simulink model "TDPBehaviourSim"  (R2020b)
settings: Solver=VariableStepAuto  StartTime=0.0  StopTime=200  FixedStep=sampleTime  RelTol=1e-3  EnableMultiTasking=on
values from neighbouring files (symbols this model uses):
  angThresh = pi/16    (= 0.196349540849)    [GameParameters.m]
  attackerKickSpeed = 0.3    [GameParameters.m]
  AwayFormation1 = [9.5 4 pi ... (first row only)    [FormationPoses.m]    (also in GameParameters.m)
  ballAngleNoise = pi/24    (= 0.1308996939)    [GameParameters.m]
  ballThresh = playerRadius + 0.03    (= 0.11)    [GameParameters.m]
  ballVelNoise = 0.05    [GameParameters.m]
  distThresh = 0.1    [GameParameters.m]
  fieldCenter = [mean(fieldLimitsX) mean(fieldLimitsY)]    [GameParameters.m]
  fieldLimitsX = [1 10]    [GameParameters.m]
  fieldLimitsY = [1 7]    [GameParameters.m]
  goalPosts = [1  2.7 2 ... (first row only)    [GameParameters.m]
  HomeFormation1 = [1.5 4 0 ... (first row only)    [FormationPoses.m]    (also in GameParameters.m)
  maxSpeed = 0.1    [GameParameters.m]
  maxTurnSpeed = 0.05    [GameParameters.m]
  playerRadius = 0.08    [GameParameters.m]
  sampleTime = 0.5    [GameParameters.m]
undefined symbols (not defined in the file or in its folder): DiscIntNeverNeededParam
libraries: mobileRoboticsLib x33, soccerRobotLib x16
(part 1 of 2)
settings Model: SimulationMode=accelerator  SnapshotBufferSize=20  Creator=2683935i  LastModifiedBy=2683935i
settings SolverCC: AutoInsertRateTranBlk=on
settings DataIOCC: SaveOutput=off  SaveTime=off
settings OptimizationCC: DefaultParameterBehavior=Inlined  InlineInvariantSignals=on  EnhancedBackFolding=on  PassReuseOutputArgsAs=Individual arguments  StateBitsets=on  DataBitsets=on  ZeroExternalMemoryAtStartup=off  ZeroInternalMemoryAtStartup=off  NoFixptDivByZeroProtection=on  LifeSpan=1  OptimizeBlockOrder=speed  DifferentSizesBufferReuse=on  EfficientTunableParamExpr=on
settings DebuggingCC: ParameterTunabilityLossMsg=error  UnderSpecifiedDimensionMsg=warning
settings HardwareCC: ProdBitPerPointer=32  ProdBitPerSizeT=32  ProdBitPerPtrDiffT=32  ProdLargestAtomicFloat=None  ProdIntDivRoundTo=Floor  ProdWordSize=32  ProdHWDeviceType=Generic->Custom
settings SFSimCC: MATLABDynamicMemAlloc=off
settings RTWCC: Description=Embedded Coder  SystemTargetFile=ert.tlc  TLCOptions=-p0  GenCodeOnly=on  TemplateMakefile=ert_default_tmf  GenerateReport=on  RTWVerbose=off  IncludeHyperlinkInReport=on  LaunchReport=on
settings CodeAppCC: ForceParamTrailComments=on  IgnoreCustomStorageClasses=off  OperatorAnnotations=on  SimulinkDataObjDesc=on  SFDataObjDesc=on  CustomSymbolStrGlobalVar=rt$N$M  CustomSymbolStrType=$N$M  CustomSymbolStrFcn=$N$M$F  CustomSymbolStrMacro=$N$M  InsertBlockDesc=on
settings ERTTargetCC: TargetLangStandard=C99 (ISO)  GenerateSampleERTMain=on  IncludeMdlTerminateFcn=off  SuppressErrorStatus=on  SupportAbsoluteTime=off  PurelyIntegerCode=on  SupportNonFinite=off  SupportComplex=off  InlinedParameterPlacement=NonHierarchical  RootIOFormat=Structure reference  ERTCustomFileTemplate=example_file_process.tlc

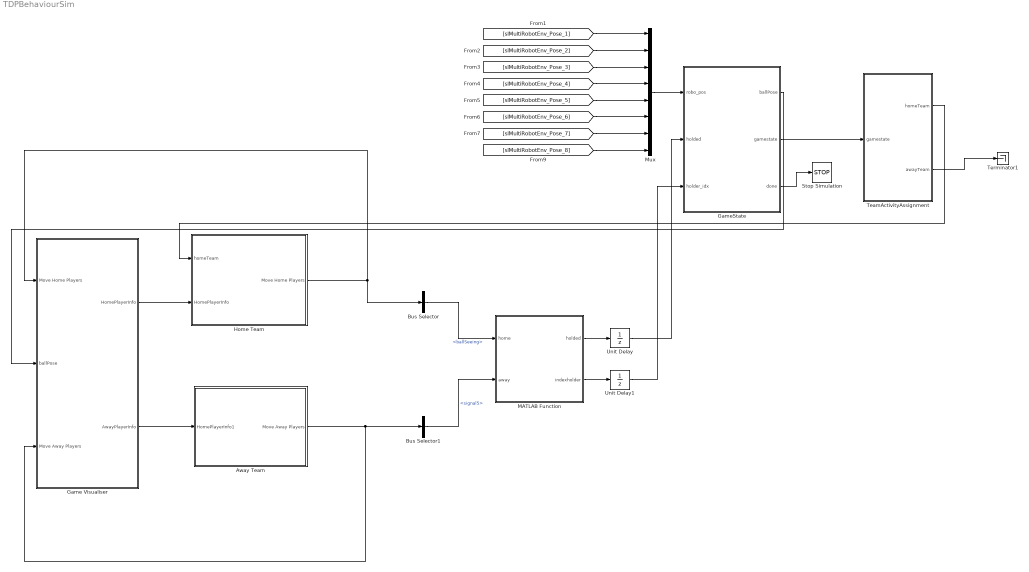
== system TDPBehaviourSim ==
  Away Team : Subsystem
  Bus Selector : BusSelector  OutputSignals=ballSeeing
  Bus Selector1 : BusSelector  OutputSignals=signal5
  Game Visualiser : Subsystem
  GameState : Stateflow chart  TreatAsAtomicUnit=on
  Home Team : Subsystem
  MATLAB Function : MATLAB Function  TreatAsAtomicUnit=on
  Mux : Mux  Inputs=8
  Stop Simulation : Stop
  TeamActivityAssignment : Stateflow chart  TreatAsAtomicUnit=on
  Terminator1 : Terminator
  Unit Delay : UnitDelay  SampleTime=-1  HasFrameUpgradeWarning=on
  Unit Delay1 : UnitDelay  SampleTime=-1  HasFrameUpgradeWarning=on
  wires:
  Home Team/1(Move Home Players) -> Bus Selector/1, Game Visualiser/1(Move Home Players)
  Away Team/1(Move Away Players) -> Game Visualiser/3(Move Away Players), Bus Selector1/1
  Game Visualiser/1(HomePlayerInfo) -> Home Team/2(HomePlayerInfo)
  Game Visualiser/2(AwayPlayerInfo) -> Away Team/1(HomePlayerInfo1)
  [slMultiRobotEnv_Pose_4] -> Mux/4
  [slMultiRobotEnv_Pose_8] -> Mux/8
  [slMultiRobotEnv_Pose_1] -> Mux/1
  Mux/1 -> GameState/1(robo_pos)
  [slMultiRobotEnv_Pose_2] -> Mux/2
  [slMultiRobotEnv_Pose_3] -> Mux/3
  GameState/1(ballPose) -> Game Visualiser/2(ballPose)
  TeamActivityAssignment/2(awayTeam) -> Terminator1/1
  TeamActivityAssignment/1(homeTeam) -> Home Team/1(homeTeam)
  Bus Selector/1 -> MATLAB Function/1(home)  "<ballSeeing>"
  Bus Selector1/1 -> MATLAB Function/2(away)  "<signal5>"
  GameState/3(done) -> Stop Simulation/1
  [slMultiRobotEnv_Pose_5] -> Mux/5
  [slMultiRobotEnv_Pose_6] -> Mux/6
  [slMultiRobotEnv_Pose_7] -> Mux/7
  GameState/2(gamestate) -> TeamActivityAssignment/1(gamestate)
  MATLAB Function/2(indexholder) -> Unit Delay1/1
  Unit Delay1/1 -> GameState/3(holder_idx)
  MATLAB Function/1(holded) -> Unit Delay/1
  Unit Delay/1 -> GameState/2(holded)

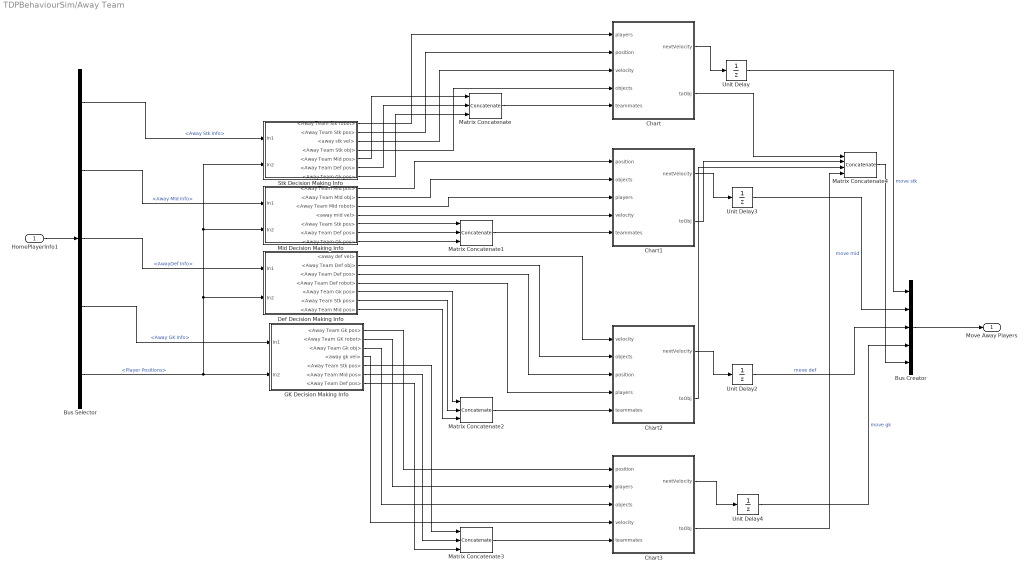
== system TDPBehaviourSim/Away Team ==
  HomePlayerInfo1 : Inport
  Bus Creator : BusCreator  Inputs=5
  Bus Selector : BusSelector  OutputSignals=Away Stk Info,Away MId Info,AwayDef Info,Away GK Info,Player Positions
  Chart : Stateflow chart  TreatAsAtomicUnit=on
      settings: PortSchema="{\"entries\":[{\"content\":{\"sides\":[{\"content\":{\"connectorIds\":[\"In3\",\"In1\",\"In2\",\"In5\",\"In4\"]},\"type\":\"ConnectorPlacement.EquallySpacedRectSide\",\"uuid\":\"cf890ef0-0ec1-422c-ab9c-1628c873ebf0\"},{\"content\":{\"connectorIds\":[\"Out1\",\"Out2\"],\"side\":\"RIGHT\"},\"type\":\"ConnectorPlacement.EquallySpacedRectSide\",\"uuid\":\"0000e457-9393-40de-9950-8ff794b83dda\"},{\"content\":{\"connectorIds\":[],\"side\":\"TOP\"},\"type\":\"ConnectorPlacement.EquallySpacedRectSide\",\"uuid\":\"7dd8e30a-3952-4d7c-b255-0e0c48dee19a\"}]},\"type\":\"ConnectorPlacement.EquallySpacedConnector\",\"uuid\":\"e8168788-1535-41f0-a84f-110f92e839bd\"}],\"packageUris\":[\"http://schema.mathworks.com/mf0/Connector/R2020b\"],\"version\":\"1.0\"}"
  Chart1 : Stateflow chart  TreatAsAtomicUnit=on
      settings: PortSchema="{\"entries\":[{\"content\":{\"sides\":[{\"content\":{\"connectorIds\":[\"In1\",\"In5\",\"In3\",\"In2\",\"In4\"]},\"type\":\"ConnectorPlacement.EquallySpacedRectSide\",\"uuid\":\"cf890ef0-0ec1-422c-ab9c-1628c873ebf0\"},{\"content\":{\"connectorIds\":[\"Out1\",\"Out2\"],\"side\":\"RIGHT\"},\"type\":\"ConnectorPlacement.EquallySpacedRectSide\",\"uuid\":\"0000e457-9393-40de-9950-8ff794b83dda\"},{\"content\":{\"connectorIds\":[],\"side\":\"TOP\"},\"type\":\"ConnectorPlacement.EquallySpacedRectSide\",\"uuid\":\"7dd8e30a-3952-4d7c-b255-0e0c48dee19a\"}]},\"type\":\"ConnectorPlacement.EquallySpacedConnector\",\"uuid\":\"e8168788-1535-41f0-a84f-110f92e839bd\"}],\"packageUris\":[\"http://schema.mathworks.com/mf0/Connector/R2020b\"],\"version\":\"1.0\"}"
  Chart2 : Stateflow chart  TreatAsAtomicUnit=on
      settings: PortSchema="{\"entries\":[{\"content\":{\"sides\":[{\"content\":{\"connectorIds\":[\"In2\",\"In5\",\"In1\",\"In3\",\"In4\"]},\"type\":\"ConnectorPlacement.EquallySpacedRectSide\",\"uuid\":\"cf890ef0-0ec1-422c-ab9c-1628c873ebf0\"},{\"content\":{\"connectorIds\":[\"Out1\",\"Out2\"],\"side\":\"RIGHT\"},\"type\":\"ConnectorPlacement.EquallySpacedRectSide\",\"uuid\":\"0000e457-9393-40de-9950-8ff794b83dda\"},{\"content\":{\"connectorIds\":[],\"side\":\"TOP\"},\"type\":\"ConnectorPlacement.EquallySpacedRectSide\",\"uuid\":\"7dd8e30a-3952-4d7c-b255-0e0c48dee19a\"}]},\"type\":\"ConnectorPlacement.EquallySpacedConnector\",\"uuid\":\"e8168788-1535-41f0-a84f-110f92e839bd\"}],\"packageUris\":[\"http://schema.mathworks.com/mf0/Connector/R2020b\"],\"version\":\"1.0\"}"
  Chart3 : Stateflow chart  TreatAsAtomicUnit=on
      settings: PortSchema="{\"entries\":[{\"content\":{\"sides\":[{\"content\":{\"connectorIds\":[\"In1\",\"In3\",\"In5\",\"In2\",\"In4\"]},\"type\":\"ConnectorPlacement.EquallySpacedRectSide\",\"uuid\":\"cf890ef0-0ec1-422c-ab9c-1628c873ebf0\"},{\"content\":{\"connectorIds\":[\"Out1\",\"Out2\"],\"side\":\"RIGHT\"},\"type\":\"ConnectorPlacement.EquallySpacedRectSide\",\"uuid\":\"0000e457-9393-40de-9950-8ff794b83dda\"},{\"content\":{\"connectorIds\":[],\"side\":\"TOP\"},\"type\":\"ConnectorPlacement.EquallySpacedRectSide\",\"uuid\":\"7dd8e30a-3952-4d7c-b255-0e0c48dee19a\"}]},\"type\":\"ConnectorPlacement.EquallySpacedConnector\",\"uuid\":\"e8168788-1535-41f0-a84f-110f92e839bd\"}],\"packageUris\":[\"http://schema.mathworks.com/mf0/Connector/R2020b\"],\"version\":\"1.0\"}"
  Def Decision Making Info : Subsystem
  GK Decision Making Info : Subsystem
  Matrix Concatenate{,1..3} (4 alike) : Concatenate  NumInputs=3  Mode=Multidimensional array  ConcatenateDimension=2
  Matrix Concatenate4 : Concatenate  NumInputs=4  Mode=Multidimensional array
  Mid Decision Making Info : Subsystem
  Stk Decision Making Info : Subsystem
  Unit Delay{,2..4} (4 alike) : UnitDelay  SampleTime=-1  HasFrameUpgradeWarning=on
  Move Away Players : Outport
  wires:
  Def Decision Making Info/7(<Away Team Mid pos>) -> Matrix Concatenate2/3
  Def Decision Making Info/6(<Away Team Stk pos>) -> Matrix Concatenate2/2
  Def Decision Making Info/3(<Away Team Def pos>) -> Chart2/1(position)
  Matrix Concatenate3/1 -> Chart3/4(teammates)
  Unit Delay/1 -> Bus Creator/1  "move stk"
  Stk Decision Making Info/6(<Away Team Def pos>) -> Matrix Concatenate/2
  Stk Decision Making Info/5(<Away Team Mid pos>) -> Matrix Concatenate/1
  Mid Decision Making Info/6(<Away Team Def pos>) -> Matrix Concatenate1/2
  Def Decision Making Info/1(<away def vel>) -> Chart2/2(velocity)
  Mid Decision Making Info/1(<Away Team Mid pos>) -> Chart1/1(position)
  Mid Decision Making Info/7(<Away Team Gk pos>) -> Matrix Concatenate1/3
  Mid Decision Making Info/4(<away mid vel>) -> Chart1/2(velocity)
  GK Decision Making Info/7(<Away Team Def pos>) -> Matrix Concatenate3/3
  GK Decision Making Info/2(<Away Team GK robot>) -> Chart3/3(players)
  GK Decision Making Info/1(<Away Team Gk pos>) -> Chart3/1(position)
  Matrix Concatenate/1 -> Chart/4(teammates)
  Stk Decision Making Info/4(<Away Team Stk obj>) -> Chart/5(objects)
  Chart1/1(nextVelocity) -> Unit Delay3/1
  Mid Decision Making Info/2(<Away Team MId obj>) -> Chart1/5(objects)
  Chart2/1(nextVelocity) -> Unit Delay2/1
  Mid Decision Making Info/3(<Away Team MId robot>) -> Chart1/3(players)
  GK Decision Making Info/6(<Away Team Mid pos>) -> Matrix Concatenate3/2
  Chart/1(nextVelocity) -> Unit Delay/1
  Unit Delay4/1 -> Bus Creator/4  "move gk"
  Mid Decision Making Info/5(<Away Team Stk pos>) -> Matrix Concatenate1/1
  Def Decision Making Info/2(<Away Team Def obj>) -> Chart2/5(objects)
  Stk Decision Making Info/1(<Away Team Stk robot>) -> Chart/3(players)
  Def Decision Making Info/4(<Away Team Def robot>) -> Chart2/3(players)
  Chart3/1(nextVelocity) -> Unit Delay4/1
  Matrix Concatenate1/1 -> Chart1/4(teammates)
  GK Decision Making Info/3(<Away Team Gk obj>) -> Chart3/5(objects)
  Stk Decision Making Info/3(<away stk vel>) -> Chart/2(velocity)
  GK Decision Making Info/4(<away gk vel>) -> Chart3/2(velocity)
  Stk Decision Making Info/2(<Away Team Stk pos>) -> Chart/1(position)
  Matrix Concatenate2/1 -> Chart2/4(teammates)
  Stk Decision Making Info/7(<Away Team Gk pos>) -> Matrix Concatenate/3
  Def Decision Making Info/5(<Away Team Gk pos>) -> Matrix Concatenate2/1
  Unit Delay2/1 -> Bus Creator/3  "move def"
  GK Decision Making Info/5(<Away Team Stk pos>) -> Matrix Concatenate3/1
  Unit Delay3/1 -> Bus Creator/2  "move mid"
  Bus Creator/1 -> Move Away Players/1
  HomePlayerInfo1/1 -> Bus Selector/1
  Bus Selector/5 -> Stk Decision Making Info/2(In2), Mid Decision Making Info/2(In2), Def Decision Making Info/2(In2), GK Decision Making Info/2(In2)  "<Player Positions>"
  Bus Selector/1 -> Stk Decision Making Info/1(In1)  "<Away Stk Info>"
  Bus Selector/2 -> Mid Decision Making Info/1(In1)  "<Away MId Info>"
  Bus Selector/3 -> Def Decision Making Info/1(In1)  "<AwayDef Info>"
  Bus Selector/4 -> GK Decision Making Info/1(In1)  "<Away GK Info>"
  Chart/2(toObj) -> Matrix Concatenate4/1
  Chart1/2(toObj) -> Matrix Concatenate4/2
  Chart2/2(toObj) -> Matrix Concatenate4/3
  Chart3/2(toObj) -> Matrix Concatenate4/4
  Matrix Concatenate4/1 -> Bus Creator/5

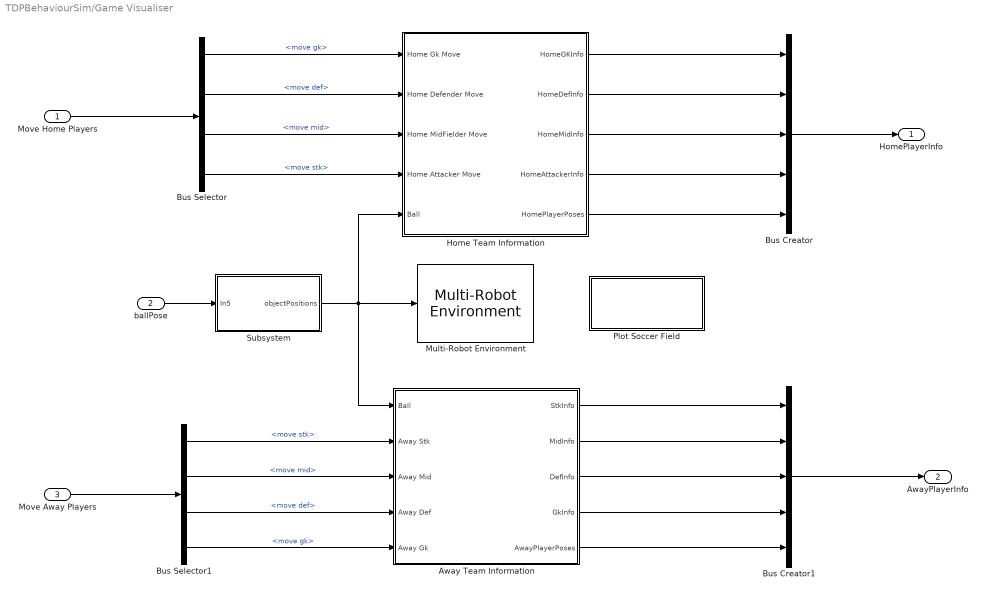
== system TDPBehaviourSim/Game Visualiser ==
  Move Home Players : Inport
  ballPose : Inport  Port=2
  Move Away Players : Inport  Port=3
  Away Team Information : Subsystem
  Bus Creator : BusCreator  Inputs=5
  Bus Creator1 : BusCreator  Inputs=5
  Bus Selector : BusSelector  OutputSignals=move gk,move def,move mid,move stk
  Bus Selector1 : BusSelector  OutputSignals=move stk,move mid,move def,move gk
  Home Team Information : Subsystem
  Multi-Robot Environment : mobileRoboticsLib/Environments/Multi-Robot Environment  numRobots=numPlayers  mapName=map  showWaypoints=off  showObjects=on  objectColors=objColors  objectMarkers='o^^^^'  showRobotIds=on  plotSensorLines=off
      settings: SourceProductName=Mobile Robotics Simulation Toolbox
  Plot Soccer Field : MATLAB Function  TreatAsAtomicUnit=on
  Subsystem : Subsystem
  HomePlayerInfo : Outport
  AwayPlayerInfo : Outport  Port=2
  wires:
  Home Team Information/1(HomeGKInfo) -> Bus Creator/1
  Home Team Information/2(HomeDefInfo) -> Bus Creator/2
  Home Team Information/3(HomeMidInfo) -> Bus Creator/3
  Home Team Information/4(HomeAttackerInfo) -> Bus Creator/4
  Home Team Information/5(HomePlayerPoses) -> Bus Creator/5
  Away Team Information/1(StkInfo) -> Bus Creator1/1
  Away Team Information/2(MidInfo) -> Bus Creator1/2
  Away Team Information/3(DefInfo) -> Bus Creator1/3
  Away Team Information/4(GkInfo) -> Bus Creator1/4
  Away Team Information/5(AwayPlayerPoses) -> Bus Creator1/5
  Subsystem/1(objectPositions) -> Multi-Robot Environment/1, Away Team Information/1(Ball), Home Team Information/5(Ball)
  ballPose/1 -> Subsystem/1(In5)
  Move Home Players/1 -> Bus Selector/1
  Bus Selector/1 -> Home Team Information/1(Home Gk Move)  "<move gk>"
  Bus Selector/2 -> Home Team Information/2(Home Defender Move)  "<move def>"
  Bus Selector/3 -> Home Team Information/3(Home MidFielder Move)  "<move mid>"
  Bus Selector/4 -> Home Team Information/4(Home Attacker Move)  "<move stk>"
  Move Away Players/1 -> Bus Selector1/1
  Bus Selector1/4 -> Away Team Information/5("Away Gk ")  "<move gk>"
  Bus Selector1/3 -> Away Team Information/4(Away Def)  "<move def>"
  Bus Selector1/2 -> Away Team Information/3(Away Mid)  "<move mid>"
  Bus Selector1/1 -> Away Team Information/2(Away Stk)  "<move stk>"
  Bus Creator/1 -> HomePlayerInfo/1
  Bus Creator1/1 -> AwayPlayerInfo/1

== system TDPBehaviourSim/GameState/BallDynamics.InBounds.BallFree ==
  Action Port : ActionPort
      settings: CopyFcn=Stateflow.SLINSF.SimulinkMan.removeBlockPreDeleteFcn  PreDeleteFcn=Stateflow.SLINSF.SimulinkMan.unsafePredeleteFcn
  Gain : Gain  Gain=-0.25
  Position Integrator : DiscreteIntegrator  InitialCondition=fieldCenter  SampleTime=-1  StateName=ballPos  ICPrevOutput=DiscIntNeverNeededParam  ICPrevScaledInput=DiscIntNeverNeededParam
  Signal Specification : SignalSpecification  Dimensions=[1 2]
  Velocity Integrator : DiscreteIntegrator  InitialCondition=[0 0]  SampleTime=-1  StateName=ballVel  ICPrevOutput=DiscIntNeverNeededParam  ICPrevScaledInput=DiscIntNeverNeededParam
  ballPose : Outport  VectorParamsAs1DForOutWhenUnconnected=off
  wires:
  Gain/1 -> Velocity Integrator/1
  Velocity Integrator/1 -> Signal Specification/1
  Position Integrator/1 -> ballPose/1
  Signal Specification/1 -> Position Integrator/1, Gain/1

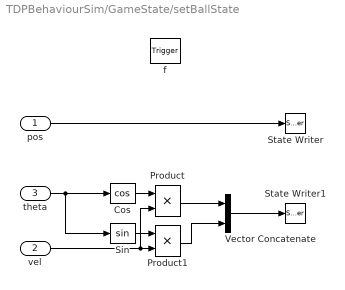
== system TDPBehaviourSim/GameState/setBallState ==
  pos : Inport  OutDataTypeStr=double  PortDimensions=[1 2]
  vel : Inport  Port=2  OutDataTypeStr=double  PortDimensions=1
  theta : Inport  Port=3  OutDataTypeStr=double  PortDimensions=1
  f : TriggerPort  TriggerType=function-call  VariantControl=(inherit)
      settings: CopyFcn=Stateflow.SLINSF.SimulinkMan.removeBlockPreDeleteFcn  PreDeleteFcn=Stateflow.SLINSF.SimulinkMan.unsafePredeleteFcn
  Cos : Trigonometry  Operator=cos
  Product : Product
  Product1 : Product
  Sin : Trigonometry
  State Writer : StateWriter  StateOwnerBlock=../../BallDynamics.InBounds.BallFree/Position Integrator  StateName=ballPos
  State Writer1 : StateWriter  StateOwnerBlock=../../BallDynamics.InBounds.BallFree/Velocity Integrator  StateName=ballVel
  Vector Concatenate : Concatenate  Mode=Multidimensional array  ConcatenateDimension=2
  wires:
  Vector Concatenate/1 -> State Writer1/1
  Product1/1 -> Vector Concatenate/2
  Product/1 -> Vector Concatenate/1
  theta/1 -> Cos/1, Sin/1
  Sin/1 -> Product1/1
  vel/1 -> Product1/2, Product/2
  Cos/1 -> Product/1
  pos/1 -> State Writer/1

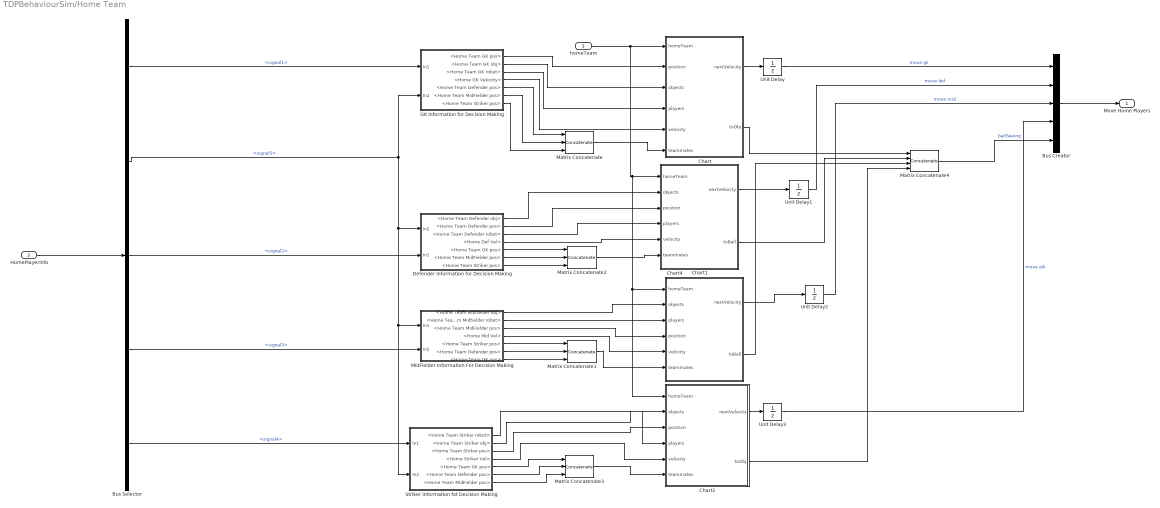
== system TDPBehaviourSim/Home Team ==
  homeTeam : Inport
  HomePlayerInfo : Inport  Port=2
  Bus Creator : BusCreator  Inputs=5
  Bus Selector : BusSelector  OutputSignals=signal1,signal5,signal2,signal3,signal4
  Chart : Stateflow chart  TreatAsAtomicUnit=on
      settings: PortSchema="{\"entries\":[{\"content\":{\"sides\":[{\"content\":{\"connectorIds\":[\"In1\",\"In2\",\"In6\",\"In4\",\"In3\",\"In5\"]},\"type\":\"ConnectorPlacement.EquallySpacedRectSide\",\"uuid\":\"cf890ef0-0ec1-422c-ab9c-1628c873ebf0\"},{\"content\":{\"connectorIds\":[\"Out1\",\"Out2\"],\"side\":\"RIGHT\"},\"type\":\"ConnectorPlacement.EquallySpacedRectSide\",\"uuid\":\"0000e457-9393-40de-9950-8ff794b83dda\"},{\"content\":{\"connectorIds\":[],\"side\":\"TOP\"},\"type\":\"ConnectorPlacement.EquallySpacedRectSide\",\"uuid\":\"7dd8e30a-3952-4d7c-b255-0e0c48dee19a\"}]},\"type\":\"ConnectorPlacement.EquallySpacedConnector\",\"uuid\":\"e8168788-1535-41f0-a84f-110f92e839bd\"}],\"packageUris\":[\"http://schema.mathworks.com/mf0/Connector/R2020b\"],\"version\":\"1.0\"}"
  Chart1 : Stateflow chart  TreatAsAtomicUnit=on
      settings: PortSchema="{\"entries\":[{\"content\":{\"sides\":[{\"content\":{\"connectorIds\":[\"In1\",\"In6\",\"In2\",\"In4\",\"In3\",\"In5\"]},\"type\":\"ConnectorPlacement.EquallySpacedRectSide\",\"uuid\":\"cf890ef0-0ec1-422c-ab9c-1628c873ebf0\"},{\"content\":{\"connectorIds\":[\"Out1\",\"Out2\"],\"side\":\"RIGHT\"},\"type\":\"ConnectorPlacement.EquallySpacedRectSide\",\"uuid\":\"0000e457-9393-40de-9950-8ff794b83dda\"},{\"content\":{\"connectorIds\":[],\"side\":\"TOP\"},\"type\":\"ConnectorPlacement.EquallySpacedRectSide\",\"uuid\":\"7dd8e30a-3952-4d7c-b255-0e0c48dee19a\"}]},\"type\":\"ConnectorPlacement.EquallySpacedConnector\",\"uuid\":\"e8168788-1535-41f0-a84f-110f92e839bd\"}],\"packageUris\":[\"http://schema.mathworks.com/mf0/Connector/R2020b\"],\"version\":\"1.0\"}"
  Chart2 : Stateflow chart  TreatAsAtomicUnit=on
      settings: PortSchema="{\"entries\":[{\"content\":{\"sides\":[{\"content\":{\"connectorIds\":[\"In1\",\"In6\",\"In2\",\"In4\",\"In3\",\"In5\"]},\"type\":\"ConnectorPlacement.EquallySpacedRectSide\",\"uuid\":\"cf890ef0-0ec1-422c-ab9c-1628c873ebf0\"},{\"content\":{\"connectorIds\":[\"Out1\",\"Out2\"],\"side\":\"RIGHT\"},\"type\":\"ConnectorPlacement.EquallySpacedRectSide\",\"uuid\":\"0000e457-9393-40de-9950-8ff794b83dda\"},{\"content\":{\"connectorIds\":[],\"side\":\"TOP\"},\"type\":\"ConnectorPlacement.EquallySpacedRectSide\",\"uuid\":\"7dd8e30a-3952-4d7c-b255-0e0c48dee19a\"}]},\"type\":\"ConnectorPlacement.EquallySpacedConnector\",\"uuid\":\"e8168788-1535-41f0-a84f-110f92e839bd\"}],\"packageUris\":[\"http://schema.mathworks.com/mf0/Connector/R2020b\"],\"version\":\"1.0\"}"
  Chart4 : Stateflow chart  TreatAsAtomicUnit=on
      settings: PortSchema="{\"entries\":[{\"content\":{\"sides\":[{\"content\":{\"connectorIds\":[\"In1\",\"In6\",\"In4\",\"In2\",\"In3\",\"In5\"]},\"type\":\"ConnectorPlacement.EquallySpacedRectSide\",\"uuid\":\"cf890ef0-0ec1-422c-ab9c-1628c873ebf0\"},{\"content\":{\"connectorIds\":[\"Out1\",\"Out2\"],\"side\":\"RIGHT\"},\"type\":\"ConnectorPlacement.EquallySpacedRectSide\",\"uuid\":\"0000e457-9393-40de-9950-8ff794b83dda\"},{\"content\":{\"connectorIds\":[],\"side\":\"TOP\"},\"type\":\"ConnectorPlacement.EquallySpacedRectSide\",\"uuid\":\"7dd8e30a-3952-4d7c-b255-0e0c48dee19a\"}]},\"type\":\"ConnectorPlacement.EquallySpacedConnector\",\"uuid\":\"e8168788-1535-41f0-a84f-110f92e839bd\"}],\"packageUris\":[\"http://schema.mathworks.com/mf0/Connector/R2020b\"],\"version\":\"1.0\"}"
  "Defender Information for Decision Making " : Subsystem
  GK Information for Decision Making : Subsystem
  Matrix Concatenate{,1..3} (4 alike) : Concatenate  NumInputs=3  Mode=Multidimensional array  ConcatenateDimension=2
  Matrix Concatenate4 : Concatenate  NumInputs=4  Mode=Multidimensional array
  MidFielder Information For Decision Making : Subsystem
  Striker Information fot Decision Making : Subsystem
  Unit Delay{,1..3} (4 alike) : UnitDelay  SampleTime=-1  HasFrameUpgradeWarning=on
  Move Home Players : Outport
  wires:
  "Defender Information for Decision Making "/7(<Home Team Striker pos>) -> Matrix Concatenate2/3
  Matrix Concatenate1/1 -> Chart4/5(teammates)
  Striker Information fot Decision Making/7(<Home Team MidFielder pos>) -> Matrix Concatenate3/3
  "Defender Information for Decision Making "/3(<Home Team Defender robot>) -> Chart1/4(players)
  GK Information for Decision Making/1(<Home Team GK pos>) -> Chart/2(position)
  GK Information for Decision Making/4(<Home GK Velocity>) -> Chart/3(velocity)
  Chart/1(nextVelocity) -> Unit Delay/1
  "Defender Information for Decision Making "/6(<Home Team MidFielder pos>) -> Matrix Concatenate2/2
  GK Information for Decision Making/7(<Home Team Striker pos>) -> Matrix Concatenate/3
  MidFielder Information For Decision Making/3(<Home Team MidFielder pos>) -> Chart4/2(position)
  GK Information for Decision Making/3(<Home Team GK robot>) -> Chart/4(players)
  "Defender Information for Decision Making "/1(<Home Team Defender obj>) -> Chart1/6(objects)
  "Defender Information for Decision Making "/4(<Home Def Vel>) -> Chart1/3(velocity)
  GK Information for Decision Making/5(<Home Team Defender pos>) -> Matrix Concatenate/1
  MidFielder Information For Decision Making/2(<Home Team Midfielder robot>) -> Chart4/4(players)
  GK Information for Decision Making/6(<Home Team MidFielder pos>) -> Matrix Concatenate/2
  Matrix Concatenate2/1 -> Chart1/5(teammates)
  Striker Information fot Decision Making/6(<Home Team Defender pos>) -> Matrix Concatenate3/2
  MidFielder Information For Decision Making/5(<Home Team Striker pos>) -> Matrix Concatenate1/1
  MidFielder Information For Decision Making/7(<Home Team GK pos>) -> Matrix Concatenate1/3
  GK Information for Decision Making/2(<Home Team GK obj>) -> Chart/6(objects)
  MidFielder Information For Decision Making/4(<Home Mid Vel>) -> Chart4/3(velocity)
  MidFielder Information For Decision Making/1(<Home Team Midfielder obj>) -> Chart4/6(objects)
  Striker Information fot Decision Making/5(<Home Team GK pos>) -> Matrix Concatenate3/1
  Unit Delay/1 -> Bus Creator/1  "move gk"
  MidFielder Information For Decision Making/6(<Home Team Defender pos>) -> Matrix Concatenate1/2
  "Defender Information for Decision Making "/2(<Home Team Defender pos>) -> Chart1/2(position)
  "Defender Information for Decision Making "/5(<Home Team GK pos>) -> Matrix Concatenate2/1
  Chart2/1(nextVelocity) -> Unit Delay3/1
  Unit Delay2/1 -> Bus Creator/3  "move mid"
  Unit Delay1/1 -> Bus Creator/2  "move def"
  Matrix Concatenate/1 -> Chart/5(teammates)
  Bus Creator/1 -> Move Home Players/1
  HomePlayerInfo/1 -> Bus Selector/1
  Bus Selector/1 -> GK Information for Decision Making/1(In1)  "<signal1>"
  Bus Selector/2 -> Striker Information fot Decision Making/2(In2), MidFielder Information For Decision Making/1(In1), "Defender Information for Decision Making "/1(In2), GK Information for Decision Making/2(In2)  "<signal5>"
  Bus Selector/3 -> "Defender Information for Decision Making "/2(In1)  "<signal2>"
  Bus Selector/4 -> MidFielder Information For Decision Making/2(In2)  "<signal3>"
  Bus Selector/5 -> Striker Information fot Decision Making/1(In1)  "<signal4>"
  Chart/2(toObj) -> Matrix Concatenate4/1
  Chart2/2(toObj) -> Matrix Concatenate4/4
  Unit Delay3/1 -> Bus Creator/4  "move stk"
  Matrix Concatenate4/1 -> Bus Creator/5  "ballSeeing"
  Striker Information fot Decision Making/3(<Home Team Striker pos>) -> Chart2/2(position)
  Striker Information fot Decision Making/1(<Home Team Striker robot>) -> Chart2/4(players)
  Striker Information fot Decision Making/2(<Home Team Striker obj>) -> Chart2/6(objects)
  Striker Information fot Decision Making/4(<Home Striker Vel>) -> Chart2/3(velocity)
  Matrix Concatenate3/1 -> Chart2/5(teammates)
  Chart1/2(toBall) -> Matrix Concatenate4/2
  Chart1/1(nextVelocity) -> Unit Delay1/1
  Chart4/1(nextVelocity) -> Unit Delay2/1
  Chart4/2(toBall) -> Matrix Concatenate4/3
  homeTeam/1 -> Chart2/1(homeTeam), Chart4/1(homeTeam), Chart1/1(homeTeam), Chart/1(homeTeam)

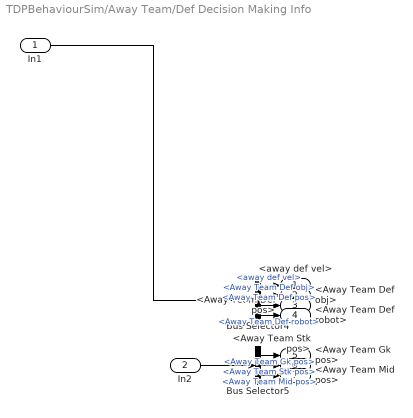
== system TDPBehaviourSim/Away Team/Def Decision Making Info ==
  In1 : Inport
  In2 : Inport  Port=2
  Bus Selector4 : BusSelector  OutputSignals=away def vel,Away Team Def obj,Away Team Def pos,Away Team Def robot
  Bus Selector5 : BusSelector  OutputSignals=Away Team Gk pos,Away Team Stk pos,Away Team Mid pos
  <away def vel> : Outport
  <Away Team Def obj> : Outport  Port=2
  <Away Team Def pos> : Outport  Port=3
  <Away Team Def robot> : Outport  Port=4
  <Away Team Gk pos> : Outport  Port=5
  <Away Team Stk pos> : Outport  Port=6
  <Away Team Mid pos> : Outport  Port=7
  wires:
  Bus Selector5/2 -> <Away Team Stk pos>/1  "<Away Team Stk pos>"
  Bus Selector5/3 -> <Away Team Mid pos>/1  "<Away Team Mid pos>"
  Bus Selector4/2 -> <Away Team Def obj>/1  "<Away Team Def obj>"
  Bus Selector4/3 -> <Away Team Def pos>/1  "<Away Team Def pos>"
  Bus Selector4/1 -> <away def vel>/1  "<away def vel>"
  In2/1 -> Bus Selector5/1
  In1/1 -> Bus Selector4/1
  Bus Selector4/4 -> <Away Team Def robot>/1  "<Away Team Def robot>"
  Bus Selector5/1 -> <Away Team Gk pos>/1  "<Away Team Gk pos>"

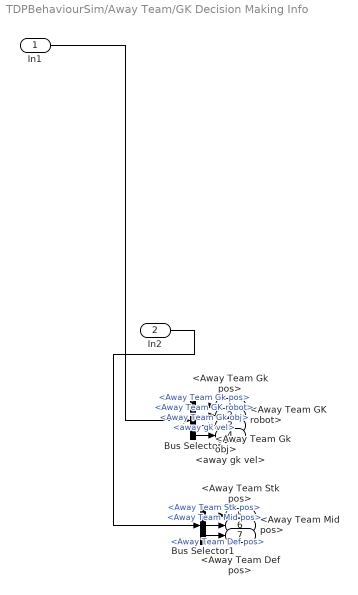
== system TDPBehaviourSim/Away Team/GK Decision Making Info ==
  In1 : Inport
  In2 : Inport  Port=2
  Bus Selector : BusSelector  OutputSignals=Away Team Gk pos,Away Team GK robot,Away Team Gk obj,away gk vel
  Bus Selector1 : BusSelector  OutputSignals=Away Team Stk pos,Away Team Mid pos,Away Team Def pos
  <Away Team Gk pos> : Outport
  <Away Team GK robot> : Outport  Port=2
  <Away Team Gk obj> : Outport  Port=3
  <away gk vel> : Outport  Port=4
  <Away Team Stk pos> : Outport  Port=5
  <Away Team Mid pos> : Outport  Port=6
  <Away Team Def pos> : Outport  Port=7
  wires:
  In2/1 -> Bus Selector1/1
  Bus Selector/2 -> <Away Team GK robot>/1  "<Away Team GK robot>"
  Bus Selector/3 -> <Away Team Gk obj>/1  "<Away Team Gk obj>"
  In1/1 -> Bus Selector/1
  Bus Selector1/3 -> <Away Team Def pos>/1  "<Away Team Def pos>"
  Bus Selector/1 -> <Away Team Gk pos>/1  "<Away Team Gk pos>"
  Bus Selector1/1 -> <Away Team Stk pos>/1  "<Away Team Stk pos>"
  Bus Selector/4 -> <away gk vel>/1  "<away gk vel>"
  Bus Selector1/2 -> <Away Team Mid pos>/1  "<Away Team Mid pos>"

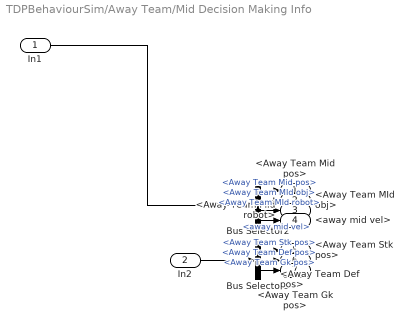
== system TDPBehaviourSim/Away Team/Mid Decision Making Info ==
  In1 : Inport
  In2 : Inport  Port=2
  Bus Selector2 : BusSelector  OutputSignals=Away Team Mid pos,Away Team MId obj,Away Team MId robot,away mid vel
  Bus Selector3 : BusSelector  OutputSignals=Away Team Stk pos,Away Team Def pos,Away Team Gk pos
  <Away Team Mid pos> : Outport
  <Away Team MId obj> : Outport  Port=2
  <Away Team MId robot> : Outport  Port=3
  <away mid vel> : Outport  Port=4
  <Away Team Stk pos> : Outport  Port=5
  <Away Team Def pos> : Outport  Port=6
  <Away Team Gk pos> : Outport  Port=7
  wires:
  Bus Selector2/2 -> <Away Team MId obj>/1  "<Away Team MId obj>"
  Bus Selector3/1 -> <Away Team Stk pos>/1  "<Away Team Stk pos>"
  Bus Selector2/3 -> <Away Team MId robot>/1  "<Away Team MId robot>"
  In1/1 -> Bus Selector2/1
  Bus Selector3/2 -> <Away Team Def pos>/1  "<Away Team Def pos>"
  Bus Selector3/3 -> <Away Team Gk pos>/1  "<Away Team Gk pos>"
  In2/1 -> Bus Selector3/1
  Bus Selector2/1 -> <Away Team Mid pos>/1  "<Away Team Mid pos>"
  Bus Selector2/4 -> <away mid vel>/1  "<away mid vel>"

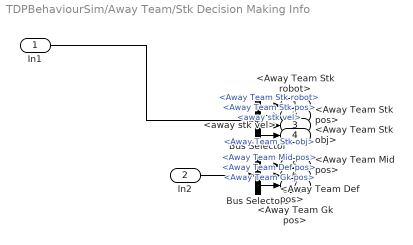
== system TDPBehaviourSim/Away Team/Stk Decision Making Info ==
  In1 : Inport
  In2 : Inport  Port=2
  Bus Selector : BusSelector  OutputSignals=Away Team Stk robot,Away Team Stk pos,away stk vel,Away Team Stk obj
  Bus Selector1 : BusSelector  OutputSignals=Away Team Mid pos,Away Team Def pos,Away Team Gk pos
  <Away Team Stk robot> : Outport
  <Away Team Stk pos> : Outport  Port=2
  <away stk vel> : Outport  Port=3
  <Away Team Stk obj> : Outport  Port=4
  <Away Team Mid pos> : Outport  Port=5
  <Away Team Def pos> : Outport  Port=6
  <Away Team Gk pos> : Outport  Port=7
  wires:
  In2/1 -> Bus Selector1/1
  Bus Selector/3 -> <away stk vel>/1  "<away stk vel>"
  Bus Selector1/2 -> <Away Team Def pos>/1  "<Away Team Def pos>"
  Bus Selector/4 -> <Away Team Stk obj>/1  "<Away Team Stk obj>"
  Bus Selector1/3 -> <Away Team Gk pos>/1  "<Away Team Gk pos>"
  Bus Selector/1 -> <Away Team Stk robot>/1  "<Away Team Stk robot>"
  Bus Selector1/1 -> <Away Team Mid pos>/1  "<Away Team Mid pos>"
  Bus Selector/2 -> <Away Team Stk pos>/1  "<Away Team Stk pos>"
  In1/1 -> Bus Selector/1

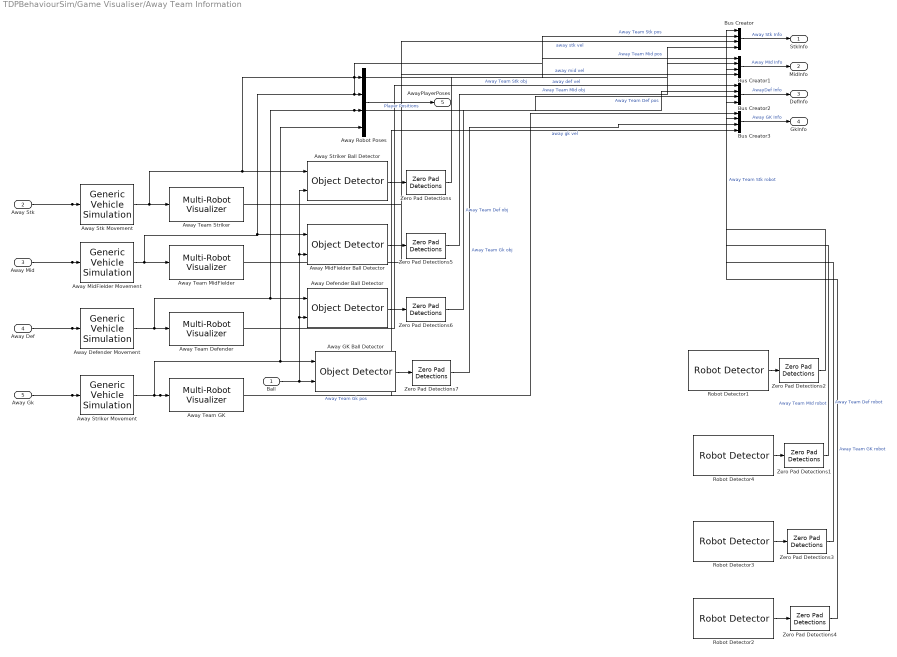
== system TDPBehaviourSim/Game Visualiser/Away Team Information ==
  Ball : Inport
  Away Stk : Inport  Port=2
  Away Mid : Inport  Port=3
  Away Def : Inport  Port=4
  "Away Gk " : Inport  Port=5
  Away Defender Ball Detector : mobileRoboticsLib/Environments/Object Detector  mapName=map  sensorOffset=objDetectorOffset  sensorAngle=objDetectorAngle  fieldOfView=objDetectorFOV  maxRange=objDetectorRange  maxDetections=objDetectorMaxHits  sampleTime=sampleTime
      settings: SourceProductName=Mobile Robotics Simulation Toolbox
  Away Defender Movement : mobileRoboticsLib/Utilities/Generic Vehicle Simulation  initX=AwayFormation1(2,1)  initY=AwayFormation1(2,2)  initAngle=AwayFormation1(2,3)  Ts=sampleTime
      settings: SourceProductName=Mobile Robotics Simulation Toolbox
  Away GK Ball Detector : mobileRoboticsLib/Environments/Object Detector  mapName=map  sensorOffset=objDetectorOffset  sensorAngle=objDetectorAngle  fieldOfView=objDetectorFOV  maxRange=objDetectorRange  maxDetections=objDetectorMaxHits  sampleTime=sampleTime
      settings: SourceProductName=Mobile Robotics Simulation Toolbox
  Away MidFielder Ball Detector : mobileRoboticsLib/Environments/Object Detector  mapName=map  sensorOffset=objDetectorOffset  sensorAngle=objDetectorAngle  fieldOfView=objDetectorFOV  maxRange=objDetectorRange  maxDetections=objDetectorMaxHits  sampleTime=sampleTime
      settings: SourceProductName=Mobile Robotics Simulation Toolbox
  Away MidFielder Movement : mobileRoboticsLib/Utilities/Generic Vehicle Simulation  initX=AwayFormation1(3,1)  initY=AwayFormation1(3,2)  initAngle=AwayFormation1(3,3)  Ts=sampleTime
      settings: SourceProductName=Mobile Robotics Simulation Toolbox
  Away Robot Poses : BusCreator  Inputs=4
  Away Stk Movement : mobileRoboticsLib/Utilities/Generic Vehicle Simulation  initX=AwayFormation1(4,1)  initY=AwayFormation1(4,2)  initAngle=AwayFormation1(4,3)  Ts=sampleTime
      settings: SourceProductName=Mobile Robotics Simulation Toolbox
  Away Striker Ball Detector : mobileRoboticsLib/Environments/Object Detector  mapName=map  sensorOffset=objDetectorOffset  sensorAngle=objDetectorAngle  fieldOfView=objDetectorFOV  maxRange=objDetectorRange  maxDetections=objDetectorMaxHits  sampleTime=sampleTime
      settings: SourceProductName=Mobile Robotics Simulation Toolbox
  Away Striker Movement : mobileRoboticsLib/Utilities/Generic Vehicle Simulation  initX=AwayFormation1(1,1)  initY=AwayFormation1(1,2)  initAngle=AwayFormation1(1,3)  Ts=sampleTime
      settings: SourceProductName=Mobile Robotics Simulation Toolbox
  Away Team Defender : mobileRoboticsLib/Environments/Multi-Robot Visualizer  idx=7  radius=playerRadius  robotColor=awayTeamColor  showTraj=on  hasLidar=off  sensorOffset=[0,0]  scanAngles=[-pi/4 0 pi/4]  maxNumScans=0  hasObjDetector=on  objDetectorOffset=objDetectorOffset  objDetectorAngle=objDetectorAngle  objDetectorFOV=objDetectorFOV  objDetectorMaxRange=objDetectorRange  hasRobotDetector=on  robotDetectorOffset=robotDetectorOffset  robotDetectorAngle=robotDetectorAngle  robotDetectorFOV=robotDetectorFOV  robotDetectorMaxRange=robotDetectorMaxHits  robotDetectorNumDetections=0
      settings: SourceProductName=Mobile Robotics Simulation Toolbox
  Away Team GK : mobileRoboticsLib/Environments/Multi-Robot Visualizer  idx=8  radius=playerRadius  robotColor=awayGKColor  showTraj=on  hasLidar=off  sensorOffset=[0,0]  scanAngles=[-pi/4 0 pi/4]  maxNumScans=0  hasObjDetector=on  objDetectorOffset=objDetectorOffset  objDetectorAngle=objDetectorAngle  objDetectorFOV=objDetectorFOV  objDetectorMaxRange=objDetectorRange  hasRobotDetector=on  robotDetectorOffset=robotDetectorOffset  robotDetectorAngle=robotDetectorAngle  robotDetectorFOV=robotDetectorFOV  robotDetectorMaxRange=robotDetectorMaxHits  robotDetectorNumDetections=0
      settings: SourceProductName=Mobile Robotics Simulation Toolbox
  Away Team MidFielder : mobileRoboticsLib/Environments/Multi-Robot Visualizer  idx=6  radius=playerRadius  robotColor=awayTeamColor  showTraj=on  hasLidar=off  sensorOffset=[0,0]  scanAngles=[-pi/4 0 pi/4]  maxNumScans=0  hasObjDetector=on  objDetectorOffset=objDetectorOffset  objDetectorAngle=objDetectorAngle  objDetectorFOV=objDetectorFOV  objDetectorMaxRange=objDetectorRange  hasRobotDetector=on  robotDetectorOffset=robotDetectorOffset  robotDetectorAngle=robotDetectorAngle  robotDetectorFOV=robotDetectorFOV  robotDetectorMaxRange=robotDetectorMaxHits  robotDetectorNumDetections=0
      settings: SourceProductName=Mobile Robotics Simulation Toolbox
  Away Team Striker : mobileRoboticsLib/Environments/Multi-Robot Visualizer  idx=5  radius=playerRadius  robotColor=awayTeamColor  showTraj=on  hasLidar=off  sensorOffset=[0,0]  scanAngles=[-pi/4 0 pi/4]  maxNumScans=0  hasObjDetector=on  objDetectorOffset=objDetectorOffset  objDetectorAngle=objDetectorAngle  objDetectorFOV=objDetectorFOV  objDetectorMaxRange=objDetectorRange  hasRobotDetector=on  robotDetectorOffset=robotDetectorOffset  robotDetectorAngle=robotDetectorAngle  robotDetectorFOV=robotDetectorFOV  robotDetectorMaxRange=robotDetectorMaxHits  robotDetectorNumDetections=0
      settings: SourceProductName=Mobile Robotics Simulation Toolbox
  Bus Creator{,1..3} (4 alike) : BusCreator  Inputs=4
  Robot Detector1 : mobileRoboticsLib/Environments/Robot Detector  mapName=map  robotIdx=5  sensorOffset=robotDetectorOffset  sensorAngle=robotDetectorAngle  sensorFOV=robotDetectorFOV  maxRange=robotDetectorRange  maxDetections=robotDetectorMaxHits  sampleTime=sampleTime
      settings: SourceProductName=Mobile Robotics Simulation Toolbox
  Robot Detector2 : mobileRoboticsLib/Environments/Robot Detector  mapName=map  robotIdx=8  sensorOffset=robotDetectorOffset  sensorAngle=robotDetectorAngle  sensorFOV=robotDetectorFOV  maxRange=robotDetectorRange  maxDetections=robotDetectorMaxHits  sampleTime=sampleTime
      settings: SourceProductName=Mobile Robotics Simulation Toolbox
  Robot Detector3 : mobileRoboticsLib/Environments/Robot Detector  mapName=map  robotIdx=7  sensorOffset=robotDetectorOffset  sensorAngle=robotDetectorAngle  sensorFOV=robotDetectorFOV  maxRange=robotDetectorRange  maxDetections=robotDetectorMaxHits  sampleTime=sampleTime
      settings: SourceProductName=Mobile Robotics Simulation Toolbox
  Robot Detector4 : mobileRoboticsLib/Environments/Robot Detector  mapName=map  robotIdx=6  sensorOffset=robotDetectorOffset  sensorAngle=robotDetectorAngle  sensorFOV=robotDetectorFOV  maxRange=robotDetectorRange  maxDetections=robotDetectorMaxHits  sampleTime=sampleTime
      settings: SourceProductName=Mobile Robotics Simulation Toolbox
  Zero Pad Detections{,5..7} (4 alike) : soccerRobotLib/Soccer Robot Simulator/Zero Pad Detections  maxHits=objDetectorMaxHits
  Zero Pad Detections{1..4} (4 alike) : soccerRobotLib/Soccer Robot Simulator/Zero Pad Detections  maxHits=robotDetectorMaxHits
  StkInfo : Outport
  MidInfo : Outport  Port=2
  DefInfo : Outport  Port=3
  GkInfo : Outport  Port=4
  AwayPlayerPoses : Outport  Port=5
  wires:
  "Away Gk "/1 -> Bus Creator3/4, Away Striker Movement/1  "away gk vel"
  Away Def/1 -> Away Defender Movement/1, Bus Creator2/1  "away def vel"
  Ball/1 -> Away Defender Ball Detector/2, Away Striker Ball Detector/2, Away MidFielder Ball Detector/2, Away GK Ball Detector/2
  Away Striker Ball Detector/1 -> Zero Pad Detections/1
  Away Defender Ball Detector/1 -> Zero Pad Detections6/1
  Away MidFielder Ball Detector/1 -> Zero Pad Detections5/1
  Away GK Ball Detector/1 -> Zero Pad Detections7/1
  Zero Pad Detections/1 -> Bus Creator/4  "Away Team Stk obj"
  Zero Pad Detections5/1 -> Bus Creator1/2  "Away Team MId obj"
  Zero Pad Detections6/1 -> Bus Creator2/2  "Away Team Def obj"
  Zero Pad Detections7/1 -> Bus Creator3/3  "Away Team Gk obj"
  Away Striker Movement/1 -> Bus Creator3/1, Away Team GK/1, Away Robot Poses/4, Away GK Ball Detector/1  "Away Team Gk pos"
  Away MidFielder Movement/1 -> Away Team MidFielder/1, Away MidFielder Ball Detector/1, Bus Creator1/1, Away Robot Poses/2  "Away Team Mid pos"
  Away Stk Movement/1 -> Bus Creator/2, Away Robot Poses/1, Away Striker Ball Detector/1, Away Team Striker/1  "Away Team Stk pos"
  Away Defender Movement/1 -> Away Defender Ball Detector/1, Away Robot Poses/3, Bus Creator2/3, Away Team Defender/1  "Away Team Def pos"
  Zero Pad Detections1/1 -> Bus Creator1/3  "Away Team MId robot"
  Zero Pad Detections3/1 -> Bus Creator2/4  "Away Team Def robot"
  Robot Detector1/1 -> Zero Pad Detections2/1
  Robot Detector4/1 -> Zero Pad Detections1/1
  Robot Detector3/1 -> Zero Pad Detections3/1
  Robot Detector2/1 -> Zero Pad Detections4/1
  Zero Pad Detections4/1 -> Bus Creator3/2  "Away Team GK robot"
  Zero Pad Detections2/1 -> Bus Creator/1  "Away Team Stk robot"
  Away Stk/1 -> Bus Creator/3, Away Stk Movement/1  "away stk vel"
  Away Mid/1 -> Bus Creator1/4, Away MidFielder Movement/1  "away mid vel"
  Bus Creator/1 -> StkInfo/1  "Away Stk Info"
  Bus Creator1/1 -> MidInfo/1  "Away MId Info"
  Bus Creator2/1 -> DefInfo/1  "AwayDef Info"
  Bus Creator3/1 -> GkInfo/1  "Away GK Info"
  Away Robot Poses/1 -> AwayPlayerPoses/1  "Player Positions"

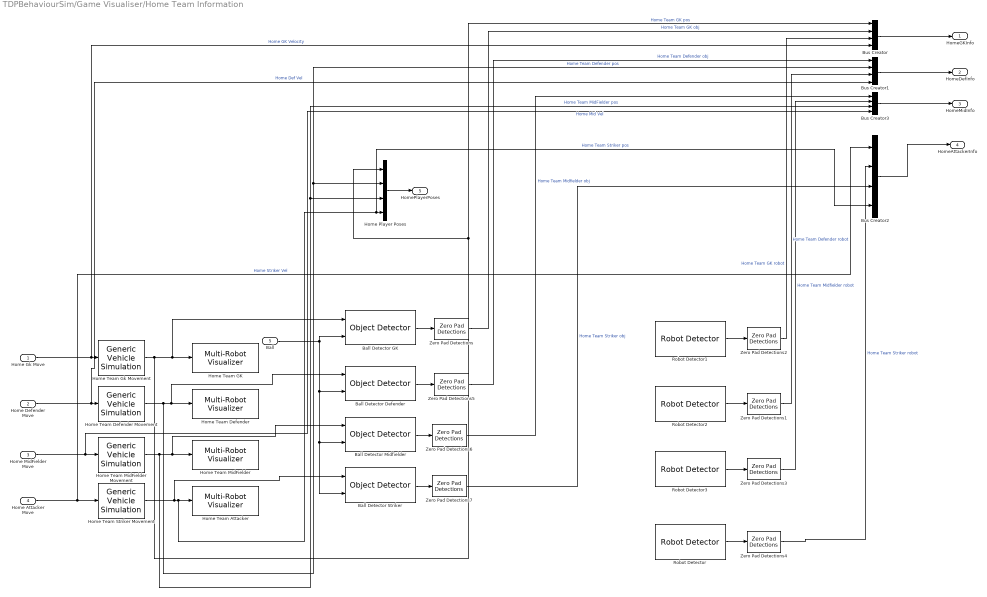
== system TDPBehaviourSim/Game Visualiser/Home Team Information ==
  Home Gk Move : Inport
  Home Defender Move : Inport  Port=2
  Home MidFielder Move : Inport  Port=3
  Home Attacker Move : Inport  Port=4
  Ball : Inport  Port=5
  Ball Detector Defender : mobileRoboticsLib/Environments/Object Detector  mapName=map  sensorOffset=objDetectorOffset  sensorAngle=objDetectorAngle  fieldOfView=objDetectorFOV  maxRange=objDetectorRange  maxDetections=objDetectorMaxHits  sampleTime=0.1
      settings: SourceProductName=Mobile Robotics Simulation Toolbox
  Ball Detector GK : mobileRoboticsLib/Environments/Object Detector  mapName=map  sensorOffset=objDetectorOffset  sensorAngle=objDetectorAngle  fieldOfView=objDetectorFOV  maxRange=objDetectorRange  maxDetections=objDetectorMaxHits  sampleTime=0.1
      settings: SourceProductName=Mobile Robotics Simulation Toolbox
  Ball Detector Midfielder : mobileRoboticsLib/Environments/Object Detector  mapName=map  sensorOffset=objDetectorOffset  sensorAngle=objDetectorAngle  fieldOfView=objDetectorFOV  maxRange=objDetectorRange  maxDetections=objDetectorMaxHits  sampleTime=0.1
      settings: SourceProductName=Mobile Robotics Simulation Toolbox
  Ball Detector Striker : mobileRoboticsLib/Environments/Object Detector  mapName=map  sensorOffset=objDetectorOffset  sensorAngle=objDetectorAngle  fieldOfView=objDetectorFOV  maxRange=objDetectorRange  maxDetections=objDetectorMaxHits  sampleTime=0.1
      settings: SourceProductName=Mobile Robotics Simulation Toolbox
  Bus Creator{,1..3} (4 alike) : BusCreator  Inputs=4
  Home Player Poses : BusCreator  Inputs=4
  Home Team Attacker : mobileRoboticsLib/Environments/Multi-Robot Visualizer  idx=4  radius=playerRadius  robotColor=homeTeamColor  showTraj=on  hasLidar=off  sensorOffset=[0,0]  scanAngles=[-pi/4 0 pi/4]  maxNumScans=0  hasObjDetector=on  objDetectorOffset=objDetectorOffset  objDetectorAngle=objDetectorAngle  objDetectorFOV=objDetectorFOV  objDetectorMaxRange=objDetectorMaxHits  hasRobotDetector=on  robotDetectorOffset=robotDetectorOffset  robotDetectorAngle=robotDetectorAngle  robotDetectorFOV=robotDetectorFOV  robotDetectorMaxRange=robotDetectorRange  robotDetectorNumDetections=0
      settings: SourceProductName=Mobile Robotics Simulation Toolbox
  Home Team Defender : mobileRoboticsLib/Environments/Multi-Robot Visualizer  idx=2  radius=playerRadius  robotColor=homeTeamColor  showTraj=on  hasLidar=off  sensorOffset=[0,0]  scanAngles=[-pi/4 0 pi/4]  maxNumScans=0  hasObjDetector=on  objDetectorOffset=objDetectorOffset  objDetectorAngle=objDetectorAngle  objDetectorFOV=objDetectorFOV  objDetectorMaxRange=objDetectorMaxHits  hasRobotDetector=off  robotDetectorOffset=[0,0]  robotDetectorAngle=0  robotDetectorFOV=pi/3  robotDetectorMaxRange=5  robotDetectorNumDetections=0
      settings: SourceProductName=Mobile Robotics Simulation Toolbox
  Home Team Defender Movement : mobileRoboticsLib/Utilities/Generic Vehicle Simulation  initX=HomeFormation1(2,1)  initY=HomeFormation1(2,2)  initAngle=HomeFormation1(2,3)  Ts=sampleTime
      settings: SourceProductName=Mobile Robotics Simulation Toolbox
  Home Team GK : mobileRoboticsLib/Environments/Multi-Robot Visualizer  idx=1  radius=playerRadius  robotColor=homeGKColor  showTraj=on  hasLidar=off  sensorOffset=[0,0]  scanAngles=[-pi/4 0 pi/4]  maxNumScans=0  hasObjDetector=on  objDetectorOffset=objDetectorOffset  objDetectorAngle=objDetectorAngle  objDetectorFOV=objDetectorFOV  objDetectorMaxRange=objDetectorRange  hasRobotDetector=on  robotDetectorOffset=robotDetectorOffset  robotDetectorAngle=robotDetectorAngle  robotDetectorFOV=robotDetectorFOV  robotDetectorMaxRange=robotDetectorRange  robotDetectorNumDetections=0
      settings: SourceProductName=Mobile Robotics Simulation Toolbox
  Home Team Gk Movement : mobileRoboticsLib/Utilities/Generic Vehicle Simulation  initX=HomeFormation1(1,1)  initY=HomeFormation1(1,2)  initAngle=HomeFormation1(1,3)  Ts=sampleTime
      settings: SourceProductName=Mobile Robotics Simulation Toolbox
  Home Team MidFielder : mobileRoboticsLib/Environments/Multi-Robot Visualizer  idx=3  radius=playerRadius  robotColor=homeTeamColor  showTraj=on  hasLidar=off  sensorOffset=[0,0]  scanAngles=[-pi/4 0 pi/4]  maxNumScans=0  hasObjDetector=off  objDetectorOffset=[0,0]  objDetectorAngle=0  objDetectorFOV=pi/3  objDetectorMaxRange=5  hasRobotDetector=off  robotDetectorOffset=[0,0]  robotDetectorAngle=0  robotDetectorFOV=pi/3  robotDetectorMaxRange=5  robotDetectorNumDetections=0
      settings: SourceProductName=Mobile Robotics Simulation Toolbox
  Home Team MidFielder Movement : mobileRoboticsLib/Utilities/Generic Vehicle Simulation  initX=HomeFormation1(3,1)  initY=HomeFormation1(3,2)  initAngle=HomeFormation1(3,3)  Ts=sampleTime
      settings: SourceProductName=Mobile Robotics Simulation Toolbox
  Home Team Striker Movement : mobileRoboticsLib/Utilities/Generic Vehicle Simulation  initX=HomeFormation1(4,1)  initY=HomeFormation1(4,2)  initAngle=HomeFormation1(4,3)  Ts=sampleTime
      settings: SourceProductName=Mobile Robotics Simulation Toolbox
  Robot Detector : mobileRoboticsLib/Environments/Robot Detector  mapName=map  robotIdx=4  sensorOffset=robotDetectorOffset  sensorAngle=robotDetectorAngle  sensorFOV=robotDetectorFOV  maxRange=robotDetectorRange  maxDetections=robotDetectorMaxHits  sampleTime=sampleTime
      settings: SourceProductName=Mobile Robotics Simulation Toolbox
  Robot Detector1 : mobileRoboticsLib/Environments/Robot Detector  mapName=map  robotIdx=1  sensorOffset=robotDetectorOffset  sensorAngle=robotDetectorAngle  sensorFOV=robotDetectorFOV  maxRange=robotDetectorRange  maxDetections=robotDetectorMaxHits  sampleTime=sampleTime
      settings: SourceProductName=Mobile Robotics Simulation Toolbox
  Robot Detector2 : mobileRoboticsLib/Environments/Robot Detector  mapName=map  robotIdx=2  sensorOffset=robotDetectorOffset  sensorAngle=robotDetectorAngle  sensorFOV=robotDetectorFOV  maxRange=robotDetectorRange  maxDetections=robotDetectorMaxHits  sampleTime=sampleTime
      settings: SourceProductName=Mobile Robotics Simulation Toolbox
  Robot Detector3 : mobileRoboticsLib/Environments/Robot Detector  mapName=map  robotIdx=3  sensorOffset=robotDetectorOffset  sensorAngle=robotDetectorAngle  sensorFOV=robotDetectorFOV  maxRange=robotDetectorRange  maxDetections=robotDetectorMaxHits  sampleTime=sampleTime
      settings: SourceProductName=Mobile Robotics Simulation Toolbox
  Zero Pad Detections{,5..7} (4 alike) : soccerRobotLib/Soccer Robot Simulator/Zero Pad Detections  maxHits=objDetectorMaxHits
  Zero Pad Detections{1..4} (4 alike) : soccerRobotLib/Soccer Robot Simulator/Zero Pad Detections  maxHits=robotDetectorMaxHits
  HomeGKInfo : Outport
  HomeDefInfo : Outport  Port=2
  HomeMidInfo : Outport  Port=3
  HomeAttackerInfo : Outport  Port=4
  HomePlayerPoses : Outport  Port=5
  wires:
  Home Gk Move/1 -> Bus Creator/4, Home Team Gk Movement/1  "Home GK Velocity"
  Home Team Striker Movement/1 -> Bus Creator2/4, Home Player Poses/4, Home Team Attacker/1, Ball Detector Striker/1  "Home Team Striker pos"
  Home Attacker Move/1 -> Bus Creator2/1, Home Team Striker Movement/1  "Home Striker Vel"
  Home Defender Move/1 -> Bus Creator1/4, Home Team Defender Movement/1  "Home Def Vel"
  Home Team Gk Movement/1 -> Ball Detector GK/1, Home Team GK/1, Bus Creator/1, Home Player Poses/1  "Home Team GK pos"
  Home Team Defender Movement/1 -> Bus Creator1/2, Home Player Poses/2, Ball Detector Defender/1, Home Team Defender/1  "Home Team Defender pos"
  Home Team MidFielder Movement/1 -> Bus Creator3/3, Home Player Poses/3, Ball Detector Midfielder/1, Home Team MidFielder/1  "Home Team MidFielder pos"
  Home MidFielder Move/1 -> Bus Creator3/4, Home Team MidFielder Movement/1  "Home Mid Vel"
  Ball/1 -> Ball Detector GK/2, Ball Detector Striker/2, Ball Detector Midfielder/2, Ball Detector Defender/2
  Ball Detector GK/1 -> Zero Pad Detections/1
  Ball Detector Midfielder/1 -> Zero Pad Detections6/1
  Ball Detector Defender/1 -> Zero Pad Detections5/1
  Ball Detector Striker/1 -> Zero Pad Detections7/1
  Robot Detector1/1 -> Zero Pad Detections2/1
  Robot Detector3/1 -> Zero Pad Detections3/1
  Robot Detector/1 -> Zero Pad Detections4/1
  Zero Pad Detections/1 -> Bus Creator/2  "Home Team GK obj"
  Zero Pad Detections2/1 -> Bus Creator/3  "Home Team GK robot"
  Zero Pad Detections1/1 -> Bus Creator1/3  "Home Team Defender robot"
  Robot Detector2/1 -> Zero Pad Detections1/1
  Zero Pad Detections3/1 -> Bus Creator3/2  "Home Team Midfielder robot"
  Zero Pad Detections4/1 -> Bus Creator2/2  "Home Team Striker robot"
  Zero Pad Detections5/1 -> Bus Creator1/1  "Home Team Defender obj"
  Zero Pad Detections6/1 -> Bus Creator3/1  "Home Team Midfielder obj"
  Zero Pad Detections7/1 -> Bus Creator2/3  "Home Team Striker obj"
  Home Player Poses/1 -> HomePlayerPoses/1
  Bus Creator/1 -> HomeGKInfo/1
  Bus Creator1/1 -> HomeDefInfo/1
  Bus Creator3/1 -> HomeMidInfo/1
  Bus Creator2/1 -> HomeAttackerInfo/1

== system TDPBehaviourSim/Game Visualiser/Subsystem ==
  In5 : Inport
  Constant1 : Constant  Value=goalPosts
  Object Matrix Creator : MATLAB Function  TreatAsAtomicUnit=on
  objectPositions : Outport
  wires:
  Constant1/1 -> Object Matrix Creator/2(goalPosts)
  In5/1 -> Object Matrix Creator/1(BallPos)
  Object Matrix Creator/1(objectPositions) -> objectPositions/1

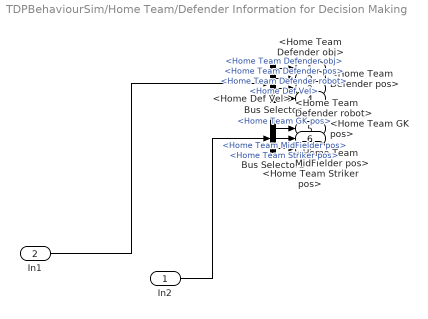
== system TDPBehaviourSim/Home Team/Defender Information for Decision Making  ==
  In2 : Inport
  In1 : Inport  Port=2
  Bus Selector : BusSelector  OutputSignals=Home Team Defender obj,Home Team Defender pos,Home Team Defender robot,Home Def Vel
  Bus Selector1 : BusSelector  OutputSignals=Home Team GK pos,Home Team MidFielder pos,Home Team Striker pos
  <Home Team Defender obj> : Outport
  <Home Team Defender pos> : Outport  Port=2
  <Home Team Defender robot> : Outport  Port=3
  <Home Def Vel> : Outport  Port=4
  <Home Team GK pos> : Outport  Port=5
  <Home Team MidFielder pos> : Outport  Port=6
  <Home Team Striker pos> : Outport  Port=7
  wires:
  In1/1 -> Bus Selector/1
  In2/1 -> Bus Selector1/1
  Bus Selector1/2 -> <Home Team MidFielder pos>/1  "<Home Team MidFielder pos>"
  Bus Selector/3 -> <Home Team Defender robot>/1  "<Home Team Defender robot>"
  Bus Selector1/1 -> <Home Team GK pos>/1  "<Home Team GK pos>"
  Bus Selector1/3 -> <Home Team Striker pos>/1  "<Home Team Striker pos>"
  Bus Selector/4 -> <Home Def Vel>/1  "<Home Def Vel>"
  Bus Selector/1 -> <Home Team Defender obj>/1  "<Home Team Defender obj>"
  Bus Selector/2 -> <Home Team Defender pos>/1  "<Home Team Defender pos>"
